simulink model "v2Drag"  (Simulink 7.8)
settings: Solver=ode45  StartTime=0.0  StopTime=10.0  RelTol=1e-3
values from neighbouring files (symbols this model uses):
  cDrag = [263.893782902 263.893782902 37.6991118431 3.15115641521e-05 3.15115641521e-05 1.28618629192e-06]    [15RunsSmallEtta.mat]    (also in 1To10withTorque.mat = [263.893782902 263.893782902 37.6991118431 0.000237563109444; 1To20Nodes.mat = [263.893782902 263.893782902 37.6991118431 0.000237563109444; 1To30HeadToTail.mat = [263.893782902 263.893782902 37.6991118431 0.000237563109444; 1To35FullFlip.mat = [263.893782902 263.893782902 37.6991118431 0.000237563109444)
settings Model: Creator=ben  LastModifiedBy=benjJohnson  TunableVars=cDrag  TunableVarsStorageClass=ImportedExtern  TunableVarsTypeQualifier=const
settings DataIOCC: SaveOutput=off  SaveTime=off
settings OptimizationCC: InlineParams=on  SimCompilerOptimization=On
settings DebuggingCC: FcnCallInpInsideContextMsg=Use local settings  StrictBusMsg=Warning

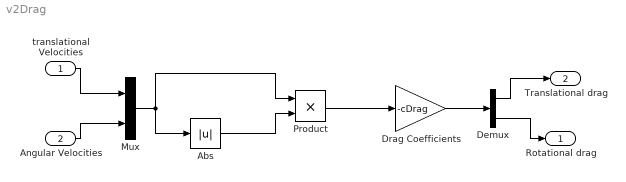
== system v2Drag ==
  translational Velocities : Inport  PortDimensions=3
  Angular Velocities : Inport  Port=2  PortDimensions=3
  Abs : Abs  ZeroCross=off
  Demux : Demux  Outputs=2
  Drag Coefficients : Gain  Gain=-cDrag
  Mux : Mux  Inputs=2
  Product : Product  RndMeth=Zero
  Rotational drag : Outport  PortDimensions=3
  Translational drag : Outport  Port=2  PortDimensions=3
  wires:
  Product/1 -> Drag Coefficients/1
  Abs/1 -> Product/2
  Mux/1 -> Abs/1, Product/1
  translational Velocities/1 -> Mux/1
  Angular Velocities/1 -> Mux/2
  Drag Coefficients/1 -> Demux/1
  Demux/1 -> Translational drag/1
  Demux/2 -> Rotational drag/1
